simulink model "SpeedSimulationTimemeresCosim"  (R2013b)
settings: Solver=FixedStepDiscrete  SolverMode=SingleTasking  StartTime=0.0  StopTime=inf  FixedStep=0.00001  RelTol=1e-3
undefined symbols (not defined in the file or in its folder): A, N
libraries: xbsIndex_r4 x2, JTAGRuntimeCosim_r4 x1
settings Model: Creator=laca  LastModifiedBy=laca

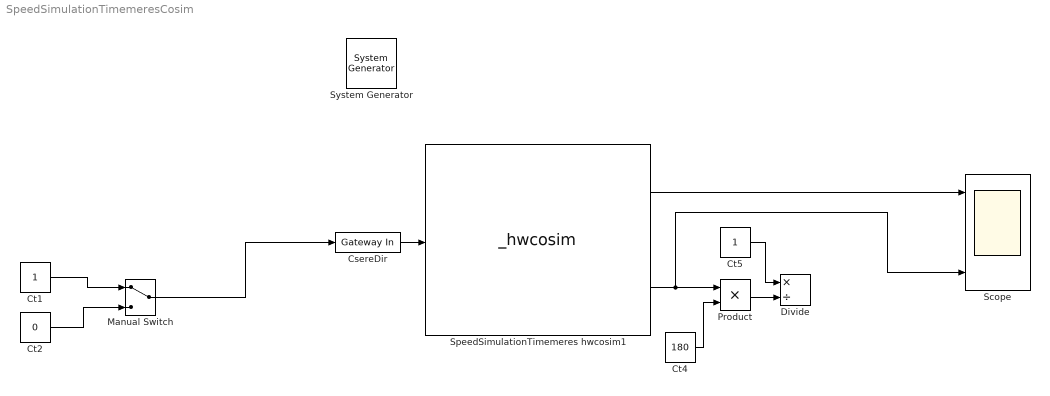
== system SpeedSimulationTimemeresCosim ==
  " System Generator" : xbsIndex_r4/ System Generator  Tag=genX  xilinxfamily=spartan3e  part=xc3s500e  speed=-4  package=pq208  synthesis_tool=XST  clock_wrapper=Clock Enables  directory=./netlist  proj_type=Project Navigator  Synth_file=XST Defaults  Impl_file=ISE Defaults  testbench=off  simulink_period=0.001  sysclk_period=20  dcm_input_clock_period=10  incr_netlist=off  trim_vbits=Everywhere in SubSystem  dbl_ovrd=According to Block Masks  core_generation=According to Block Masks  run_coregen=off  deprecated_control=off  eval_field=0  block_type=sysgen
  CsereDir : xbsIndex_r4/Gateway In  gui_display_data_type=Boolean  arith_type=Boolean  n_bits=16  bin_pt=14  preci_type=Single  exp_width=8  frac_width=24  quantization="Round  (unbiased: +/- Inf)"  overflow=Saturate  period=1  dbl_ovrd=off  timing_constraint=None  locs_specified=off  LOCs={}  UseAsADC=off  ADCChannel='1'  inherit_from_input=off  hdl_port=on  block_type=gatewayin
  Ct1 : Constant
  Ct2 : Constant  Value=0
  Ct4 : Constant  Value=180
  Ct5 : Constant
  Divide : Product  Inputs=*/
  Manual Switch : ManualSwitch
  Product : Product
  Scope : Scope  NumInputPorts=3
      settings: TickLabels=on  ShowLegends=on  TimeRange=100  YMin=-70000~-1~0  YMax=70000~1~1100
  SpeedSimulationTimemeres hwcosim1 : JTAGRuntimeCosim_r4/_hwcosim  clkSrc=Free Running  hasCombinationalPath=on  bitfileName=C:\Diak\gl\SPARTAN3E500K_slave\SystemGenrator\SebessegEsPozicio\netlist\speedsimulationtimemeres_cw.bit  skipConfig=off  cable=Auto Detect  speed=N/A  cablePort=N/A  cableLocation=Local  shareCable=off  enable_codebug=on  design_xtable=|  engineDll=JTAGCosimEngine.dll  cableWaitTime=10  bscanPos=1  IRLengths=[6,8]  useWaitBox=1  hasBufgmux=on  Scheme=Cosim  useCmdProc=1  hasProc=0  useImpact=0  printLogFile=0  block_type=jtagcosim
      | {
      |   'clkWrapper' => 'speedsimulationtimemeres_cw',
      |   'clocksGcd' => undef,
      |   'device' => 'xc3s500e-4pq208',
      |   'ports' => {
      |     'cseredir' => {
      |       'bd_port_index' => 0,
      |       'direction' => 'in',
      |       'icon_text' => 'CsereDir',
      |       'period' => 1000,
      |       'sim_pause_trigger' => false,
      |       'type' => 'Bool',
      |       'width' => 1,
      |     },
      |     'sebess_g' => {
      |       'bd_port_index' => 0,
      |       'direction' => 'out',
      |       'icon_text' => 'Sebesség',
      |       'period' => 1000,
      |       'sim_pause_trigger' => false,
      |       'type' => 'Fix_18_0',
      |       'width' => 18,
      |     },
      |     'sz_rtsebess_g1' => {
      |       'bd_port_index' => 1,
      |       'direction' => 'out',
      |       'icon_text' => 'SzürtSebesség1',
      |       'period' => 1000,
      |       'sim_pause_trigger' => false,
      |       'type' => 'UFix_16_0',
      |       'width' => 16,
      |     },
      |   },
      |   'shared_memories' => {},
      | }
  wires:
  Ct1/1 -> Manual Switch/1
  Ct2/1 -> Manual Switch/2
  Manual Switch/1 -> CsereDir/1
  CsereDir/1 -> SpeedSimulationTimemeres hwcosim1/1
  SpeedSimulationTimemeres hwcosim1/1 -> Scope/1
  SpeedSimulationTimemeres hwcosim1/2 -> Scope/3, Product/1
  Ct4/1 -> Product/2
  Product/1 -> Divide/2
  Ct5/1 -> Divide/1
